simulink model "lab6_p1"  (R2024b)
settings: Solver=ode45  StartTime=0.0  StopTime=5  MaxStep=.01  RelTol=1e-3
values from neighbouring files (symbols this model uses):
  K = 18    [lab6_p1_variables.mat]
  Kamp = 2.4    [lab6_p1_variables.mat]
  Kc = 0.4    [lab6_p1_variables.mat]
  Kpot = 1.59154943092    [lab6_p1_variables.mat]
  Tm = 0.2    [lab6_p1_variables.mat]
  Tp = 0.0108695652174    [lab6_p1_variables.mat]
  Tz = 0.434782608696    [lab6_p1_variables.mat]
settings Model: Creator=sohumb3  LastModifiedBy=sohumb3

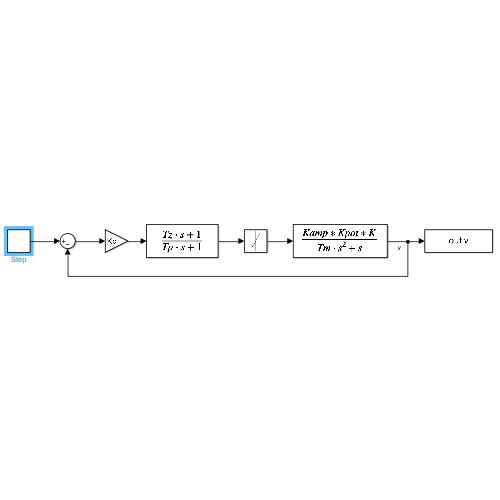
[thumbnail: Simulink's stored preview of the top-level diagram]
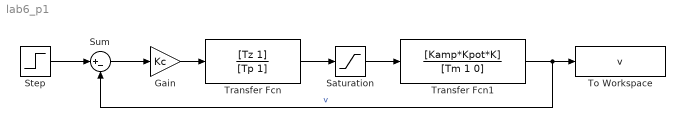
== system lab6_p1 ==
  Gain : Gain  Gain=Kc
  Saturation : Saturate  UpperLimit=10  LowerLimit=-10
  Step : Step  Time=0  After=50  SampleTime=0
  Sum : Sum  Inputs=|+-
  To Workspace : ToWorkspace  VariableName=v  SampleTime=-1
  Transfer Fcn : TransferFcn  Numerator=[Tz 1]  Denominator=[Tp 1]
  Transfer Fcn1 : TransferFcn  Numerator=[Kamp*Kpot*K]  Denominator=[Tm 1 0]
  wires:
  Transfer Fcn/1 -> Saturation/1
  Transfer Fcn1/1 -> To Workspace/1, Sum/2  "v"
  Sum/1 -> Gain/1
  Gain/1 -> Transfer Fcn/1
  Saturation/1 -> Transfer Fcn1/1
  Step/1 -> Sum/1
